simulink model "Turbo_coder"  (R2018a)
settings: Solver=VariableStepAuto  StartTime=0.0  StopTime=T  RelTol=1e-3
undefined symbols (not defined in the file): L
settings Model: Creator=vanka  LastModifiedBy=vanka

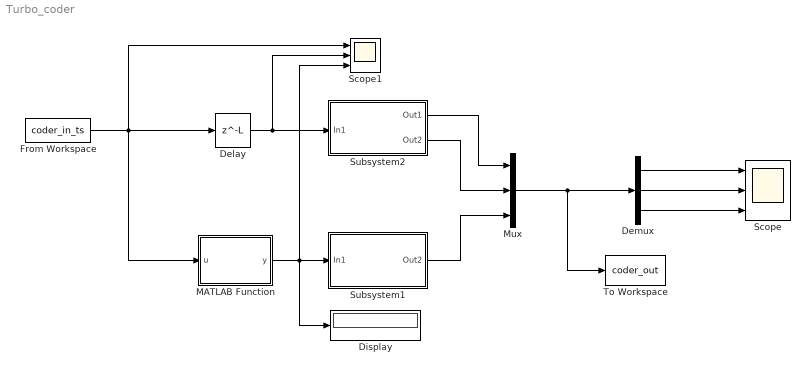
== system Turbo_coder ==
  Delay : Delay  DelayLength=L
  Demux : Demux  Outputs=3
  Display : Display
  From Workspace : FromWorkspace  VariableName=coder_in_ts  SampleTime=1  OutputAfterFinalValue=Setting to zero
  MATLAB Function : MATLAB Function  TreatAsAtomicUnit=on
  Mux : Mux  Inputs=3
  Scope : Scope  NumInputPorts=3
  Scope1 : Scope  NumInputPorts=3
  Subsystem1 : Subsystem
      mask Display: disp("RSC 1/2")
  Subsystem2 : Subsystem
      mask Display: disp("RSC 1/2")
  To Workspace : ToWorkspace  VariableName=coder_out  SaveFormat=Timeseries  SampleTime=1
  wires:
  MATLAB Function/1(y) -> Display/1, Scope1/3, Subsystem1/1(In1)
  Subsystem1/1(Out2) -> Mux/3
  Subsystem2/1(Out1) -> Mux/1
  Subsystem2/2(Out2) -> Mux/2
  Delay/1 -> Scope1/2, Subsystem2/1(In1)
  From Workspace/1 -> Scope1/1, MATLAB Function/1(u), Delay/1
  Mux/1 -> To Workspace/1, Demux/1
  Demux/2 -> Scope/2
  Demux/1 -> Scope/1
  Demux/3 -> Scope/3

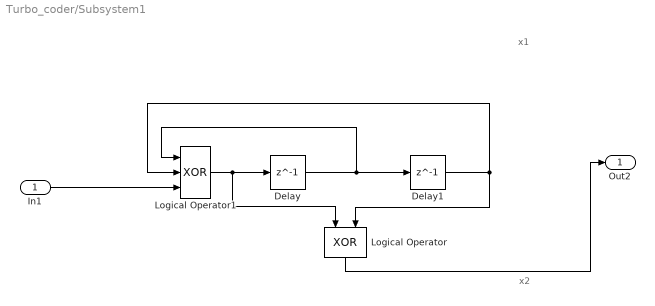
== system Turbo_coder/Subsystem1 ==
  note: x2
  note: x1
  In1 : Inport
  Delay : Delay  DelayLength=1  SampleTime=1
  Delay1 : Delay  DelayLength=1  SampleTime=1
  Logical Operator : Logic  Operator=XOR  IconShape=distinctive  AllPortsSameDT=off  OutDataTypeStr=boolean
  Logical Operator1 : Logic  Operator=XOR  Inputs=3  IconShape=distinctive  AllPortsSameDT=off  OutDataTypeStr=boolean
  Out2 : Outport
  wires:
  Logical Operator1/1 -> Logical Operator/1, Delay/1
  In1/1 -> Logical Operator1/3
  Logical Operator/1 -> Out2/1
  Delay1/1 -> Logical Operator1/2, Logical Operator/2
  Delay/1 -> Logical Operator1/1, Delay1/1

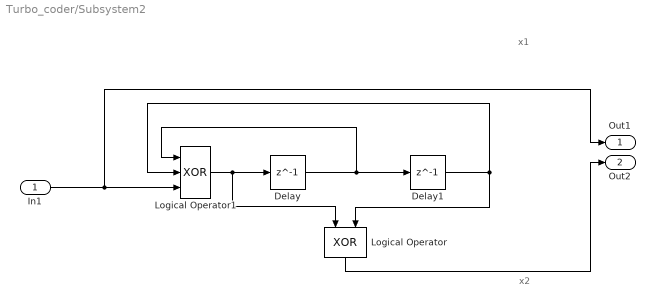
== system Turbo_coder/Subsystem2 ==
  note: x2
  note: x1
  In1 : Inport
  Delay : Delay  DelayLength=1  SampleTime=1
  Delay1 : Delay  DelayLength=1  SampleTime=1
  Logical Operator : Logic  Operator=XOR  IconShape=distinctive  AllPortsSameDT=off  OutDataTypeStr=boolean
  Logical Operator1 : Logic  Operator=XOR  Inputs=3  IconShape=distinctive  AllPortsSameDT=off  OutDataTypeStr=boolean
  Out1 : Outport
  Out2 : Outport  Port=2
  wires:
  Logical Operator1/1 -> Logical Operator/1, Delay/1
  In1/1 -> Out1/1, Logical Operator1/3
  Logical Operator/1 -> Out2/1
  Delay1/1 -> Logical Operator1/2, Logical Operator/2
  Delay/1 -> Logical Operator1/1, Delay1/1

== matlab function Turbo_coder/MATLAB Function ==
  data: u input; y output
function y = fcn(u)
%% Initial params
L = 16;
a = 3;
s = 0;
inter_table = mod((0:L-1)*a+s,L)+1;

persistent buffer interleaved_buff input_ct 
if(isempty(input_ct))
    input_ct = 0;
    buffer = zeros(1,L);
    interleaved_buff = zeros(1,L);
end


if(input_ct <= L)
    if(input_ct == L)
        input_ct = 0;
        interleaved_buff = buffer(inter_table);
    end
    
    input_ct = input_ct+1;
    buffer(input_ct) = u;
end
    y = interleaved_buff(input_ct);
